simulink model "MAVROS_Stateflow"  (R2023a)
settings: Solver=FixedStepAuto  StartTime=0.0  StopTime=1000  RelTol=1e-3
undefined symbols (not defined in the file or in its folder): CustomMode, CustomMode_SL_Info, Twist
libraries: robotlib x10, simulink x1, aerolibanimutils x1
settings Model: Creator=cesf9  LastModifiedBy=cesf9
settings OptimizationCC: EnhancedBackFolding=on  PassReuseOutputArgsAs=Individual arguments  ZeroExternalMemoryAtStartup=off  ZeroInternalMemoryAtStartup=off  MaxStackSize=64  OptimizeBlockOrder=speed  DifferentSizesBufferReuse=on  OptimizationCustomize=off  EfficientTunableParamExpr=on
settings DebuggingCC: ParameterTunabilityLossMsg=error
settings HardwareCC: ProdBitPerPointer=32  ProdBitPerSizeT=32  ProdBitPerPtrDiffT=32  ProdLargestAtomicFloat=None  ProdIntDivRoundTo=Undefined  ProdEndianess=Unspecified  ProdWordSize=32  ProdHWDeviceType=Generic->Unspecified (assume 32-bit Generic)
settings SFSimCC: MATLABDynamicMemAlloc=off
settings RTWCC: Description=Embedded Coder  SystemTargetFile=ert.tlc  HardwareBoard=Robot Operating System (ROS)  TLCOptions="-aInlineSetEventsForThisBaseRateFcn=TLC_FALSE -aSuppressMultiTaskScheduler=TLC_FALSE  -aRateBasedStepFcn=0"  TemplateMakefile=ert_default_tmf  Toolchain=Catkin  TargetLang=C++
settings CodeAppCC: ForceParamTrailComments=on  IgnoreCustomStorageClasses=off  OperatorAnnotations=on  SimulinkDataObjDesc=on  SFDataObjDesc=on  InsertBlockDesc=on

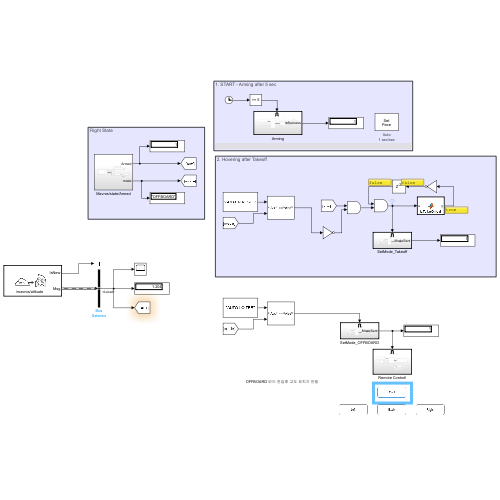
[thumbnail: Simulink's stored preview of the top-level diagram]
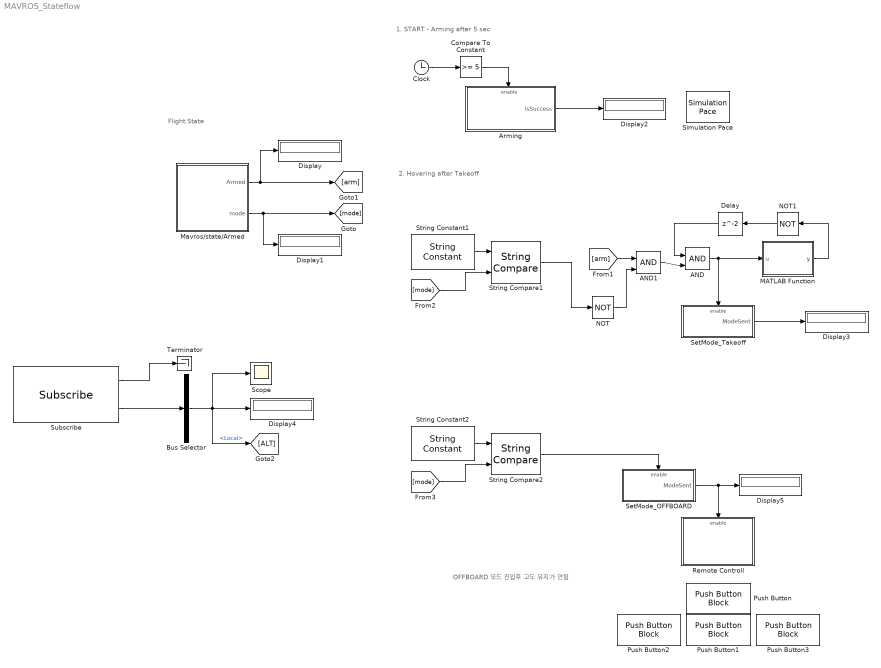
== system MAVROS_Stateflow ==
  note: OFFBOARD 모드 진입후 고도 유지가 안됨
  note: 2. Hovering after Takeoff
  note: Flight State
  note: 1. START - Arming after 5 sec
  AND : Logic  IconShape=distinctive  AllPortsSameDT=off  OutDataTypeStr=boolean
  AND1 : Logic  IconShape=distinctive  AllPortsSameDT=off  OutDataTypeStr=boolean
  Arming : Subsystem
  Bus Selector : BusSelector  OutputSignals=Local
  Clock : Clock
  Compare To Constant : simulink/Logic and Bit Operations/Compare To Constant  relop=>=  const=5  OutDataTypeStr=boolean
  Delay : Delay
  Display{,1..5} (6 alike) : Display
  MATLAB Function : MATLAB Function  TreatAsAtomicUnit=on
  Mavros/state/Armed : Subsystem
  NOT : Logic  Operator=NOT  IconShape=distinctive  AllPortsSameDT=off  OutDataTypeStr=boolean
  NOT1 : Logic  Operator=NOT  IconShape=distinctive  AllPortsSameDT=off  OutDataTypeStr=boolean
  Push Button : PushButtonBlock  ButtonText=Fwd  OffValue=0.000000
  Push Button1 : PushButtonBlock  ButtonText=Back  OffValue=0.000000
  Push Button2 : PushButtonBlock  ButtonText=Left  OffValue=0.000000
  Push Button3 : PushButtonBlock  ButtonText=Right  OffValue=0.000000
  Remote Controll : Subsystem
  Scope : Scope
  SetMode_OFFBOARD : Subsystem
  SetMode_Takeoff : Subsystem
  Simulation Pace : aerolibanimutils/Simulation Pace  SimulationPace=1  SleepMode=Auto  OutputPaceError=off  SampleTime=1/30
  String Compare1 : StringCompare
  String Compare2 : StringCompare
  String Constant1 : StringConstant  String="\"AUTO.TAKEOFF\""
  String Constant2 : StringConstant  String="\"AUTO.LOITER\""
  Subscribe : robotlib/Subscribe  topicSource=Select from ROS network  topic=/mavros/altitude  messageType=mavros_msgs/Altitude  SampleTime=-1  legacyBusStruct=off  messageQueueLength=1
  Terminator : Terminator
  wires:
  Arming/1(isSuccess) -> Display2/1
  SetMode_Takeoff/1(ModeSent) -> Display3/1
  Clock/1 -> Compare To Constant/1
  Compare To Constant/1 -> Arming/Enable
  Mavros/state/Armed/2(mode) -> Display1/1, [mode]
  Mavros/state/Armed/1(Armed) -> Display/1, [arm]
  [arm] -> AND1/1
  String Constant1/1 -> String Compare1/1
  [mode] -> String Compare1/2
  String Compare1/1 -> NOT/1
  NOT/1 -> AND1/2
  MATLAB Function/1(y) -> NOT1/1
  AND1/1 -> AND/2
  AND/1 -> MATLAB Function/1(u), SetMode_Takeoff/Enable
  NOT1/1 -> Delay/1
  Delay/1 -> AND/1
  Subscribe/1 -> Terminator/1
  Bus Selector/1 -> [ALT], Scope/1, Display4/1  "<Local>"
  Subscribe/2 -> Bus Selector/1
  String Constant2/1 -> String Compare2/1
  [mode] -> String Compare2/2
  String Compare2/1 -> SetMode_OFFBOARD/Enable
  SetMode_OFFBOARD/1(ModeSent) -> Display5/1, Remote Controll/Enable

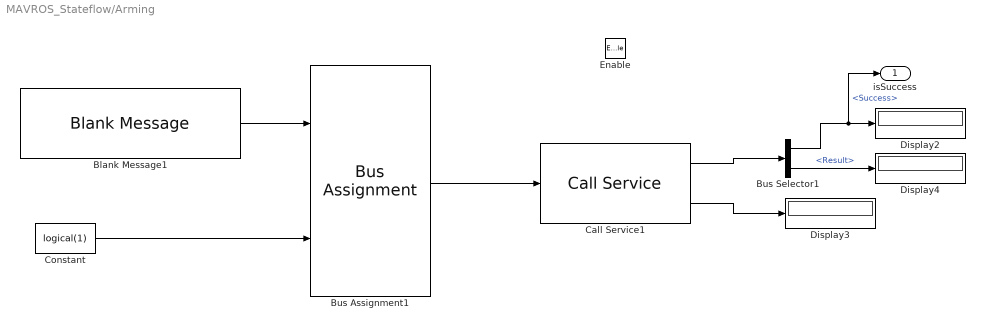
== system MAVROS_Stateflow/Arming ==
  Enable : EnablePort
  Blank Message1 : robotlib/Blank Message  messageClass=Service Request  entityType=mavros_msgs/CommandBool  messageType=mavros_msgs/CommandBoolRequest  SampleTime=inf  legacyBusStruct=off
  Bus Assignment1 : BusAssignment  AssignedSignals=Value
  Bus Selector1 : BusSelector  OutputSignals=Success,Result
  Call Service1 : robotlib/Call Service  topicSource=Select from ROS network  service=/mavros/cmd/arming  serviceType=mavros_msgs/CommandBool  connectionTimeout=5  keepPersistent=off  ShowErrorCodeOutput=on  legacyBusStruct=off
  Constant : Constant  Value=logical(1)
  Display2 : Display
  Display3 : Display
  Display4 : Display
  isSuccess : Outport
  wires:
  Bus Selector1/2 -> Display4/1  "<Result>"
  Blank Message1/1 -> Bus Assignment1/1
  Bus Assignment1/1 -> Call Service1/1
  Constant/1 -> Bus Assignment1/2
  Call Service1/1 -> Bus Selector1/1
  Bus Selector1/1 -> isSuccess/1, Display2/1  "<Success>"
  Call Service1/2 -> Display3/1

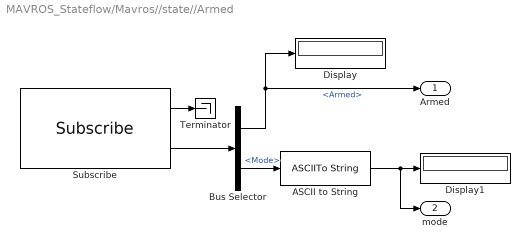
== system MAVROS_Stateflow/Mavros//state//Armed ==
  ASCII to String : ASCIIToString
  Bus Selector : BusSelector  OutputSignals=Armed,Mode
  Display : Display
  Display1 : Display
  Subscribe : robotlib/Subscribe  topicSource=Select from ROS network  topic=/mavros/state  messageType=mavros_msgs/State  SampleTime=-1  legacyBusStruct=off  messageQueueLength=1
  Terminator : Terminator
  Armed : Outport
  mode : Outport  Port=2
  wires:
  Bus Selector/2 -> ASCII to String/1  "<Mode>"
  Bus Selector/1 -> Armed/1, Display/1  "<Armed>"
  ASCII to String/1 -> mode/1, Display1/1
  Subscribe/1 -> Terminator/1
  Subscribe/2 -> Bus Selector/1

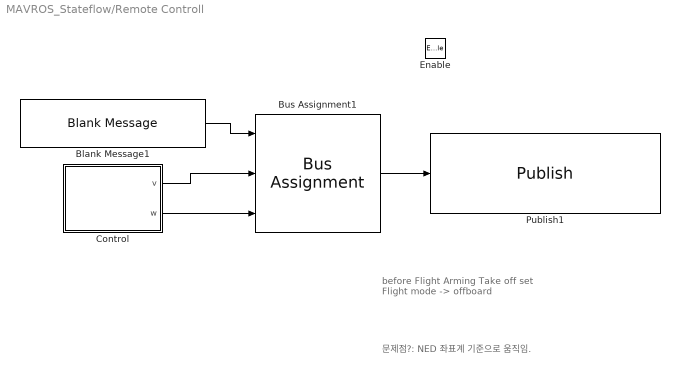
== system MAVROS_Stateflow/Remote Controll ==
  note: 문제점?: NED 좌표계 기준으로 움직임.
  note: before Flight
      | Arming
      | Take off
      | set Flight mode -> offboard
  Enable : EnablePort
  Blank Message1 : robotlib/Blank Message  messageClass=Message  entityType=geometry_msgs/TwistStamped  messageType=geometry_msgs/TwistStamped  SampleTime=0.1  legacyBusStruct=off
  Bus Assignment1 : BusAssignment  AssignedSignals=Twist.Linear.X,Twist.Angular.Z
  Control : Subsystem
  Publish1 : robotlib/Publish  topicSource=Select from ROS network  topic=/mavros/setpoint_velocity/cmd_vel  messageType=geometry_msgs/TwistStamped  legacyBusStruct=off  messageQueueLength=1
  wires:
  Bus Assignment1/1 -> Publish1/1
  Blank Message1/1 -> Bus Assignment1/1
  Control/2(w) -> Bus Assignment1/3
  Control/1(v) -> Bus Assignment1/2

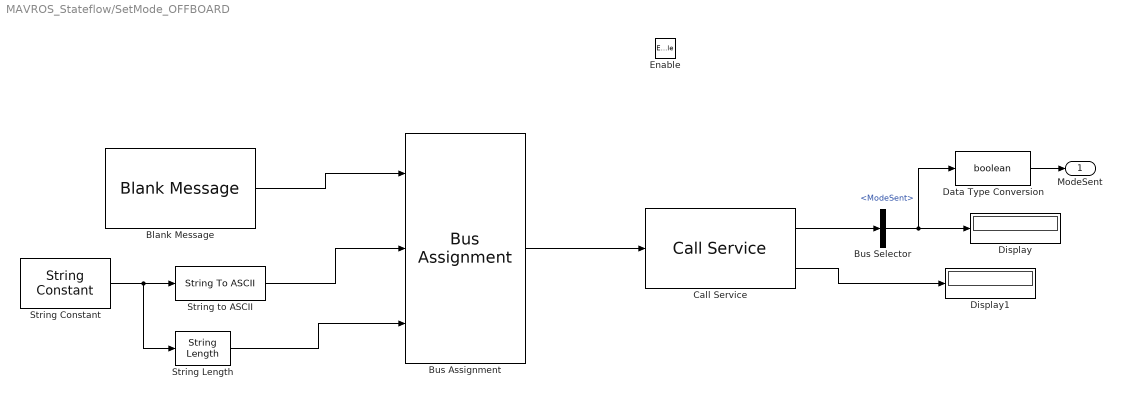
== system MAVROS_Stateflow/SetMode_OFFBOARD ==
  Enable : EnablePort
  Blank Message : robotlib/Blank Message  messageClass=Service Request  entityType=mavros_msgs/SetMode  messageType=mavros_msgs/SetModeRequest  SampleTime=inf  legacyBusStruct=off
  Bus Assignment : BusAssignment  AssignedSignals=CustomMode,CustomMode_SL_Info.CurrentLength
  Bus Selector : BusSelector  OutputSignals=ModeSent
  Call Service : robotlib/Call Service  topicSource=Select from ROS network  service=/mavros/set_mode  serviceType=mavros_msgs/SetMode  connectionTimeout=5  keepPersistent=off  ShowErrorCodeOutput=on  legacyBusStruct=off
  Data Type Conversion : DataTypeConversion  OutDataTypeStr=boolean  SaturateOnIntegerOverflow=off  RndMeth=Floor
  Display : Display
  Display1 : Display
  String Constant : StringConstant  String="\"OFFBOARD\""
  String Length : StringLength
  String to ASCII : StringToASCII  OutputVectorSize=128
  ModeSent : Outport
  wires:
  Call Service/2 -> Display1/1
  String Length/1 -> Bus Assignment/3
  Call Service/1 -> Bus Selector/1
  String to ASCII/1 -> Bus Assignment/2
  Bus Assignment/1 -> Call Service/1
  String Constant/1 -> String Length/1, String to ASCII/1
  Blank Message/1 -> Bus Assignment/1
  Bus Selector/1 -> Data Type Conversion/1, Display/1  "<ModeSent>"
  Data Type Conversion/1 -> ModeSent/1

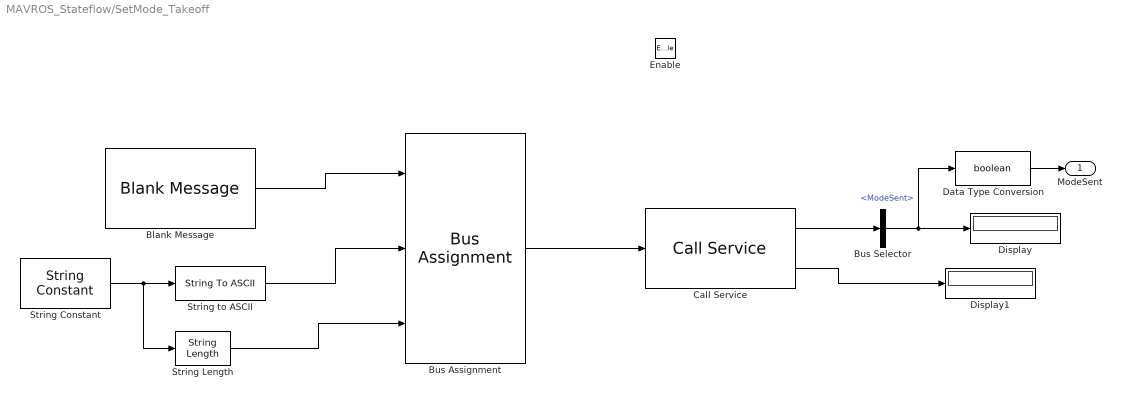
== system MAVROS_Stateflow/SetMode_Takeoff ==
  Enable : EnablePort
  Blank Message : robotlib/Blank Message  messageClass=Service Request  entityType=mavros_msgs/SetMode  messageType=mavros_msgs/SetModeRequest  SampleTime=inf  legacyBusStruct=off
  Bus Assignment : BusAssignment  AssignedSignals=CustomMode,CustomMode_SL_Info.CurrentLength
  Bus Selector : BusSelector  OutputSignals=ModeSent
  Call Service : robotlib/Call Service  topicSource=Select from ROS network  service=/mavros/set_mode  serviceType=mavros_msgs/SetMode  connectionTimeout=5  keepPersistent=off  ShowErrorCodeOutput=on  legacyBusStruct=off
  Data Type Conversion : DataTypeConversion  OutDataTypeStr=boolean  SaturateOnIntegerOverflow=off  RndMeth=Floor
  Display : Display
  Display1 : Display
  String Constant : StringConstant  String="\"AUTO.TAKEOFF\""
  String Length : StringLength
  String to ASCII : StringToASCII  OutputVectorSize=128
  ModeSent : Outport
  wires:
  Call Service/2 -> Display1/1
  String Length/1 -> Bus Assignment/3
  Call Service/1 -> Bus Selector/1
  String to ASCII/1 -> Bus Assignment/2
  Bus Assignment/1 -> Call Service/1
  String Constant/1 -> String Length/1, String to ASCII/1
  Blank Message/1 -> Bus Assignment/1
  Bus Selector/1 -> Data Type Conversion/1, Display/1  "<ModeSent>"
  Data Type Conversion/1 -> ModeSent/1

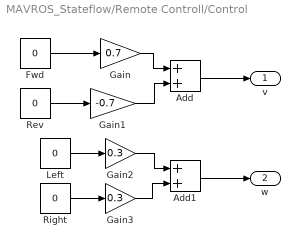
== system MAVROS_Stateflow/Remote Controll/Control ==
  Add : Sum
  Add1 : Sum
  Fwd : Constant  Value=0
  Gain : Gain  Gain=0.7
  Gain1 : Gain  Gain=-0.7
  Gain2 : Gain  Gain=0.3
  Gain3 : Gain  Gain=0.3
  Left : Constant  Value=0
  Rev : Constant  Value=0
  Right : Constant  Value=0
  v : Outport
  w : Outport  Port=2
  wires:
  Rev/1 -> Gain1/1
  Add/1 -> v/1
  Left/1 -> Gain2/1
  Fwd/1 -> Gain/1
  Right/1 -> Gain3/1
  Add1/1 -> w/1
  Gain/1 -> Add/1
  Gain1/1 -> Add/2
  Gain2/1 -> Add1/1
  Gain3/1 -> Add1/2

== matlab function MAVROS_Stateflow/MATLAB Function ==
  data: u input; y output
function y = isTakeOffed(u)
persistent takeoff

if(isempty(takeoff))
takeoff = false;
end

if(u == true)
    takeoff = true;
end

y = takeoff;
